simulink model "Project Sim"  (R2022b)
settings: Solver=FixedStepAuto  StartTime=0.0  StopTime=tspan  FixedStep=10  RelTol=1e-3
values from neighbouring files (symbols this model uses):
  E_b_ECI_0 = C2EulerAngles(C_b_ECI_0)    [A421_FinalProject_Pt5.m]    (also in A421_FinalProject_Pt6.m; Final_Project_Part_3_disturbances.m; Final_Project_Part_3_disturbances_init_Template-1.m; Final_Project_Part_3_disturbances_init_Template.m)
  J = [812.04 0 0; 0 545.37 0; 0 0 627.71]    [A421_FinalProject_Pt5.m]    (also in A421_FinalProject_Pt6.m; Final_Project_Part_3_disturbances_torques.m; Final_Project_Pt4.m; hw5.m = diag([1200, 2000, 2800]))
  q_b_ECI_0 = C2quat(C_b_ECI_0)    [A421_FinalProject_Pt5.m]    (also in A421_FinalProject_Pt6.m = [epsilon_b_ECI_0; sqrt(1-norm(epsilon_b_ECI_0)^2)]; Final_Project_Part_3_disturbances.m; Final_Project_Part_3_disturbances_init_Template-1.m; Final_Project_Part_3_disturbances_init_Template.m)
  T = [0;0;0]    [A421_FinalProject_Pt6.m]    (also in hw5.m; main.m)
  w_b_ECI_0 = [0.001; -0.001; 0.002]    [A421_FinalProject_Pt5.m]    (also in A421_FinalProject_Pt6.m; Final_Project_Part_3_disturbances.m; Final_Project_Part_3_disturbances_init_Template-1.m; Final_Project_Part_3_disturbances_init_Template.m)
settings Model: Creator=emehiel  LastModifiedBy=Jacob
settings SolverCC: AlgebraicLoopSolver=TrustRegion
settings DebuggingCC: UnconnectedInputMsg=warning  UnconnectedOutputMsg=warning  UnconnectedLineMsg=warning  SFMachineParentedDataDiag=warning
settings ModelReferenceCC: EnableRefExpFcnMdlSchedulingChecks=on

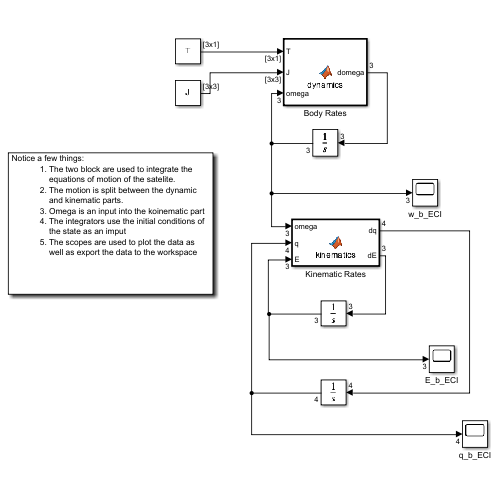
[thumbnail: Simulink's stored preview of the top-level diagram]
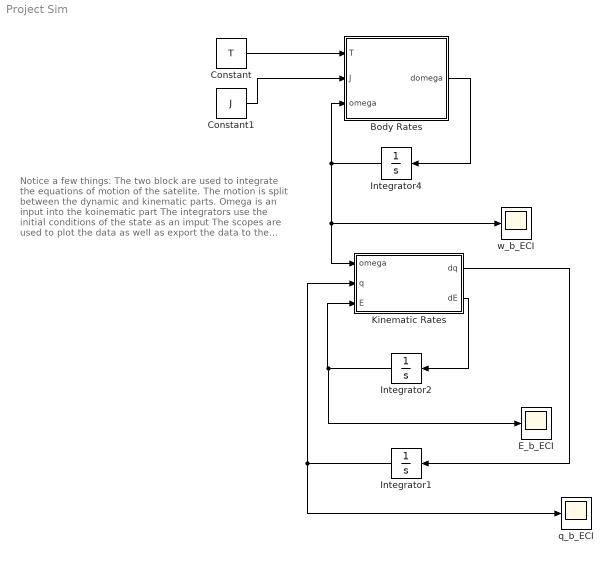
== system Project Sim ==
  note: Notice a few things:
      | The two block are used to integrate the equations of motion of the satelite.
      | The motion is split between the dynamic and kinematic parts.
      | Omega is an input into the koinematic part
      | The integrators use the initial conditions of the state as an imput
      | The scopes are used to plot the data as well as export the data to the workspace
  Body Rates : MATLAB Function  TreatAsAtomicUnit=on
  Constant : Constant  Value=T  VectorParams1D=off
  Constant1 : Constant  Value=J
  E_b_ECI : Scope
  Integrator1 : Integrator  InitialCondition=q_b_ECI_0
  Integrator2 : Integrator  InitialCondition=E_b_ECI_0
  Integrator4 : Integrator  InitialCondition=w_b_ECI_0
  Kinematic Rates : MATLAB Function  TreatAsAtomicUnit=on
  q_b_ECI : Scope
  w_b_ECI : Scope
  wires:
  Constant/1 -> Body Rates/1(T)
  Constant1/1 -> Body Rates/2(J)
  Body Rates/1(domega) -> Integrator4/1
  Integrator4/1 -> Body Rates/3(omega), w_b_ECI/1, Kinematic Rates/1(omega)
  Integrator2/1 -> E_b_ECI/1, Kinematic Rates/3(E)
  Integrator1/1 -> q_b_ECI/1, Kinematic Rates/2(q)
  Kinematic Rates/2(dE) -> Integrator2/1
  Kinematic Rates/1(dq) -> Integrator1/1

== matlab function Project Sim/Kinematic Rates ==
  data: omega input; q input; dq output; E input; dE output
function [dq,dE] = kinematics(omega, q, E)
%#codegen

I = eye(3); %Identity

% unpack quaternion
eps1 = q(1);
eps2 = q(2);
eps3 = q(3);
eps = [eps1; eps2; eps3];

eda = q(4);

% compute the derivative of the quaternion components here
             
%Quaternion rates Eq.1.56
eps_cross = [0,  -eps3, eps2;
             eps3,  0, -eps1;
             -eps2, eps1, 0];

deps = 0.5*(eda*I + eps_cross)*omega;
deda = -0.5*eps'*omega;

dq = [deps; deda];

% compute the derivative of the Euler Angle components here
            
%Euler rates
phi = E(1);
theta = E(2);
R = [1 sin(phi)*tan(theta) cos(phi)*tan(theta);
     0     cos(phi)           -sin(phi);
     0 sin(phi)*sec(theta) cos(phi)*sec(theta)];
    
dE = R*omega;


end

== matlab function Project Sim/Body Rates ==
  data: T input; J input; omega input; domega output
function domega = dynamics(T, J, omega)
%#codegen


% Compute the derivative of the angular velocity $\omega$ here

domega = J \ (T - cross(-omega, J*omega));

% phi = omega(1);
% theta = omega(2);
% psi = omega(3);
% 
% %From body to euler rates
% matrix = [1 sin(phi)*tan(theta) cos(phi)*tan(theta);
%           0    cos(phi)            -sin(phi);
%           0 sin(phi)*sec(theta) cos(phi)*sec(theta)];
% 
% domega = matrix * omega;

end
